simulink library "Radiator_basic"  (Simulink 8.2)
settings: Solver=ode45  StartTime=0.0  StopTime=10.0  RelTol=1e-3
undefined symbols (not defined in the file): A, B, C, Dd
libraries: carnot x2
settings Model: Creator=drhf  LastModifiedBy=drhf

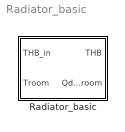
== system Radiator_basic ==
  Radiator_basic : Subsystem  mask(basic Radiator){pnomEN=1000, dtnomEN=50, expo=1.5, mcp=10*4200}
      mask prompts: pnomEN "Qdot_nom: nominal power in W"; dtnomEN "Tdiff_nom: nominal temperature difference in K"; expo "radiator exponent (> 0)"; mcp "mass * capacity per unit in J/K"
      mask help:
      | The block calculates the heat transfer of a radiator to a room according to the EN 442 equation.
      | Qdot = Qdot_nom * (Tdiff/Tdiff_nom)^n
      mask init:
      | mcap = max(1,mcp); % lower limit for capacity is 1 J/K
      | 
      | % correct values because current model 
      | % uses outlet temperature as mean temperature
      | pnom = pnomEN;
      | dtnom = dtnomEN-5;
      mask Help: web(['file:///' fullfile(path_carnot('help'),'Radiator.html')],'-helpbrowser')

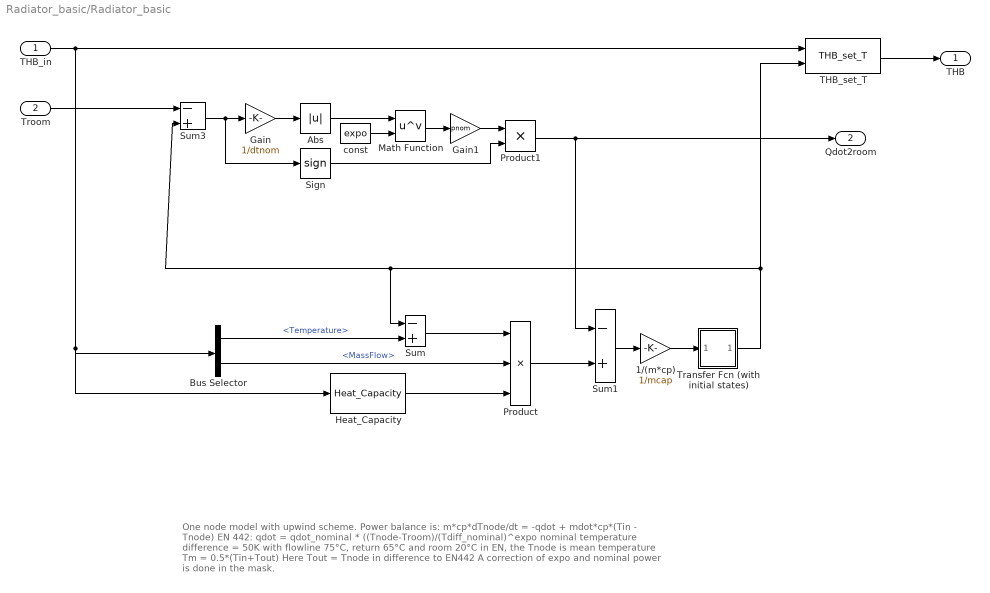
== system Radiator_basic/Radiator_basic ==
  note: One node model with upwind scheme. Power balance is:
      | m*cp*dTnode/dt = -qdot + mdot*cp*(Tin - Tnode)
      |
      | EN 442:
      | qdot = qdot_nominal * ((Tnode-Troom)/(Tdiff_nominal)^expo
      | nominal temperature difference = 50K with flowline 75°C, return 65°C and room 20°C
      | in EN, the Tnode is mean temperature Tm = 0.5*(Tin+Tout)
      |
      | Here Tout = Tnode in difference to EN442
      | A correction of expo and nominal power is done in the mask.
  THB_in : Inport
  Troom : Inport  Port=2
  1/(m*cp) : Gain  Gain=1/mcap  SaturateOnIntegerOverflow=on  OutDataTypeStr=Inherit: Same as input  ParamDataTypeStr=Inherit: Same as input
  Abs : Abs  SaturateOnIntegerOverflow=on
  Bus Selector : BusSelector  OutputSignals=Temperature,MassFlow
  Gain : Gain  Gain=1/dtnom  SaturateOnIntegerOverflow=on  OutDataTypeStr=Inherit: Same as input  ParamDataTypeStr=Inherit: Same as input
  Gain1 : Gain  Gain=pnom  SaturateOnIntegerOverflow=on  OutDataTypeStr=Inherit: Same as input  ParamDataTypeStr=Inherit: Same as input
  Heat_Capacity : carnot/Basic/Material_Properties/Heat_Capacity  SystemSampleTime=-1  VariantObject=CarlibClassic  INPUTARGUMENTS=THB  DEBUGLEVEL=DEBUGLEVEL  MAXTOTALWARNINGS=inf  MAXCONSECUTIVEWARNINGS=inf  WRITETOFILE=0  FILENAME='errors.txt'
  Math Function : Math  Operator=pow  SaturateOnIntegerOverflow=on
  Product : Product  Inputs=3  SaturateOnIntegerOverflow=on  InputSameDT=on  OutDataTypeStr=Inherit: Same as first input
  Product1 : Product  SaturateOnIntegerOverflow=on  InputSameDT=on  OutDataTypeStr=Inherit: Same as first input
  Sign : Signum
  Sum : Sum  Inputs=-+  SaturateOnIntegerOverflow=on  InputSameDT=on  OutDataTypeStr=Inherit: Same as first input
  Sum1 : Sum  Inputs=-+  SaturateOnIntegerOverflow=on  InputSameDT=on  OutDataTypeStr=Inherit: Same as first input
  Sum3 : Sum  Inputs=-+  SaturateOnIntegerOverflow=on  InputSameDT=on  OutDataTypeStr=Inherit: Same as first input
  THB_set_T : carnot/Source/Simple/THB_set_T  SystemSampleTime=-1
  Transfer Fcn (with initial states) : Subsystem  mask(Transfer Function with Initial States){N=[1], D=[1  0], X0=20}
      mask prompts: N "Numerator:"; D "Denominator:"; X0 "Initial conditions:"
      mask help: Vector expressions for numerator, and denominator. Coefficients are in descending powers of s.
      mask init:
      | [A,B,C,Dd]=tf2ss(N,D);if (isempty(X0));[m,n]=size(A);X0=zeros(1,m); end;
      mask Help: Specify the initial states for the transfer function.  The state ordering is determined by the m-file tf2ss.  There is no unique mapping of the states in a transfer function to states in a state-space representation.  However, tf2ss will consistently use the same mapping for a given transfer function.
      mask Display: dpoly(N,D,'s')
  const : Constant  Value=expo
  THB : Outport
  Qdot2room : Outport  Port=2
  wires:
  THB_in/1 -> THB_set_T/1, Heat_Capacity/1, Bus Selector/1
  THB_set_T/1 -> THB/1
  Transfer Fcn (with initial states)/1(Out1) -> THB_set_T/2, Sum/1, Sum3/2
  1/(m*cp)/1 -> Transfer Fcn (with initial states)/1(In1)
  Sum1/1 -> 1/(m*cp)/1
  Product/1 -> Sum1/2
  Heat_Capacity/1 -> Product/3
  Bus Selector/2 -> Product/2  "<MassFlow>"
  Sum/1 -> Product/1
  Product1/1 -> Sum1/1, Qdot2room/1
  const/1 -> Math Function/2
  Math Function/1 -> Gain1/1
  Gain/1 -> Abs/1
  Abs/1 -> Math Function/1
  Gain1/1 -> Product1/1
  Sum3/1 -> Gain/1, Sign/1
  Sign/1 -> Product1/2
  Bus Selector/1 -> Sum/2  "<Temperature>"
  Troom/1 -> Sum3/1

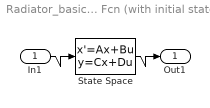
== system Radiator_basic/Radiator_basic/Transfer Fcn (with initial states) ==
  In1 : Inport
  State Space : StateSpace  A=A  B=B  C=C  D=Dd  X0=X0
  Out1 : Outport  InitialOutput=0
  wires:
  In1/1 -> State Space/1
  State Space/1 -> Out1/1
